simulink model "mdl"  (R2024a)
settings: Solver=ode1  StartTime=0.0  StopTime=inf  FixedStep=0.1  RelTol=1e-3  EnableMultiTasking=on
values from neighbouring files (symbols this model uses):
  A = 1    [init.m]
  Cw = 1.1    [init.m]
  fr = 0.02    [init.m]
  g = 9.81    [init.m]
  i1 = 74/9    (= 8.22222222222)    [init.m]
  i2 = 58/10    (= 5.8)    [init.m]
  Jachse_mitte = 0.003    [init.m]
  Jachse_unten = 0.052    [init.m]
  Jmotor = 0.001    [init.m]
  Jrad = 0.2    [init.m]
  Kp = 4000    [init.m]
  m = 455    [init.m]
  m_achse_mitte = Jachse_mitte * i2*i2 / (rR*rR)    (= 1.70347629346)    [init.m]
  m_achse_unten = Jachse_unten / (rR*rR)    (= 0.877732533291)    [init.m]
  m_motor = Jmotor * i1*i1*i2*i2 / (rR*rR)    (= 38.3878032221)    [init.m]
  m_raeder = 4 * Jrad / (rR*rR)    (= 13.5035774353)    [init.m]
  rho = 1.2    [init.m]
  rR = 0.2434    [init.m]
  stop_distance = 10.6182    [init.m]
  Tn = 200    [init.m]
undefined symbols (not defined in the file or in its folder): gradient_distance_lookup, gradient_lookup
settings Model: Creator=roustiam  LastModifiedBy=Nico Hörter
settings SolverCC: AlgebraicLoopSolver=TrustRegion
settings DataIOCC: LimitDataPoints=on  SaveFormat=Array  SignalLoggingSaveFormat=ModelDataLogs  ReturnWorkspaceOutputs=off  SignalLoggingName=sigsOut
settings OptimizationCC: BlockReduction=off  BooleanDataType=off  ExpressionDepthLimit=2147483647  InitFltsAndDblsToZero=on  LifeSpan=inf
settings DebuggingCC: SaveWithParameterizedLinksMsg=none  UnderspecifiedInitializationDetection=Classic  MergeDetectMultiDrivingBlocksExec=none  SignalResolutionControl=TryResolveAllWithWarning  MultiTaskDSMMsg=warning  MultiTaskCondExecSysMsg=none  FcnCallInpInsideContextMsg=warning  UnconnectedInputMsg=warning  UnconnectedOutputMsg=warning  UnconnectedLineMsg=warning  StateNameClashWarn=warning  SFUnexpectedBacktrackingDiag=warning  SFNoUnconditionalDefaultTransitionDiag=warning  ArithmeticOperatorsInVariantConditions=warning
settings HardwareCC: ProdBitPerPointer=32  ProdBitPerSizeT=32  ProdBitPerPtrDiffT=32  ProdLargestAtomicFloat=None  ProdIntDivRoundTo=Undefined  ProdEndianess=Unspecified  ProdWordSize=32  ProdHWDeviceType=32-bit Generic  TargetUnknown=on
settings ModelReferenceCC: EnableRefExpFcnMdlSchedulingChecks=on  PropagateSignalLabelsOutOfModel=off
settings SFSimCC: SimUseLocalCustomCode=off  CustomCodeUndefinedFunction=UseInterfaceOnly
settings RTWCC: RTWUseLocalCustomCode=off  GPUComputeCapability=3.5
settings CodeAppCC: StateflowObjectComments=on
settings GRTTargetCC: TargetFcnLib=ansi_tfl_tmw.mat  TargetLangStandard=C89/C90 (ANSI)  CombineOutputUpdateFcns=off  GRTInterface=on
settings ConfigComp: CovMetricSettings=dw  CovSaveCumulativeToWorkspaceVar=on  CovSaveSingleToWorkspaceVar=on  CovExternalEMLEnable=off

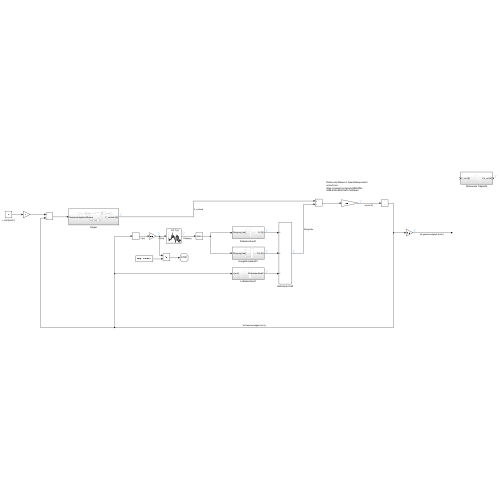
[thumbnail: Simulink's stored preview of the top-level diagram]
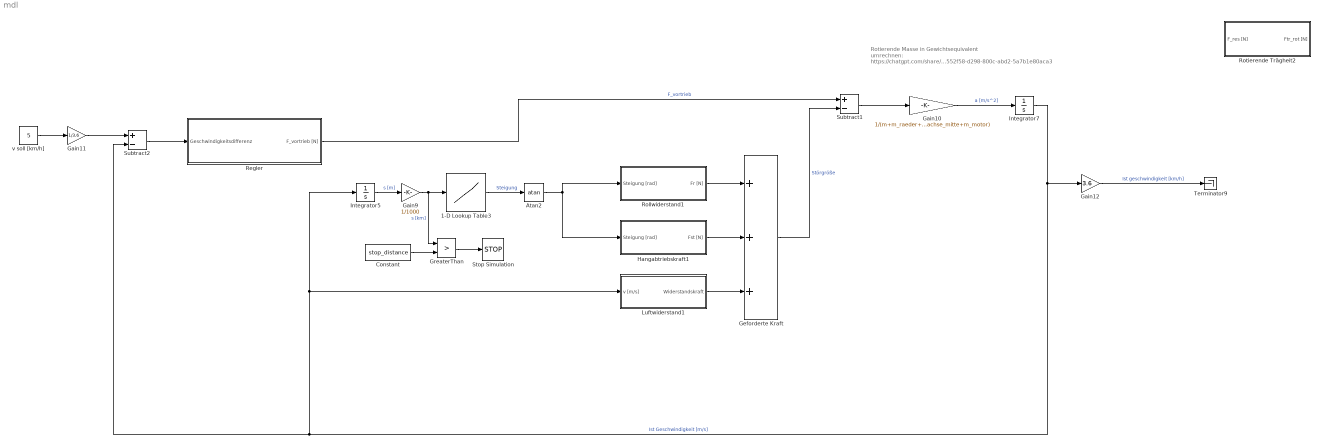
== system mdl ==
  note: Rotierende Masse in Gewichtsequivalent umrechnen:
      | https://chatgpt.com/share/68552f58-d298-800c-abd2-5a7b1e80aca3
  1-D Lookup Table3 : Lookup_n-D  NumberOfTableDimensions=1  BreakpointsForDimension1=gradient_distance_lookup  Table=gradient_lookup  ExtrapMethod=Clip  InternalRulePriority=Speed  RndMeth=Simplest
  Atan2 : Trigonometry  Operator=atan
  Constant : Constant  Value=stop_distance
  Gain10 : Gain  Gain=1/(m+m_raeder+m_achse_unten+m_achse_mitte+m_motor)
  Gain11 : Gain  Gain=1/3.6
  Gain12 : Gain  Gain=3.6
  Gain9 : Gain  Gain=1/1000
  Geforderte Kraft : Sum  Inputs=+++
  GreaterThan : RelationalOperator  Operator=>  OutDataTypeStr=boolean  RndMeth=Simplest  InputSameDT=off
  Hangabtriebskraft1 : Subsystem
  Integrator5 : Integrator
  Integrator7 : Integrator
  Luftwiderstand1 : Subsystem
  Regler : Subsystem
  Rollwiderstand1 : Subsystem
  Rotierende Trägheit2 : Subsystem
  Stop Simulation : Stop
  Subtract1 : Sum  Inputs=+-
  Subtract2 : Sum  Inputs=+-
  Terminator9 : Terminator
  v soll [km/h] : Constant  Value=5
  wires:
  Atan2/1 -> Rollwiderstand1/1(Steigung [rad]), Hangabtriebskraft1/1(Steigung [rad])
  1-D Lookup Table3/1 -> Atan2/1  "Steigung"
  Gain9/1 -> GreaterThan/1, 1-D Lookup Table3/1  "s [km]"
  Integrator5/1 -> Gain9/1  "s [m]"
  Rollwiderstand1/1(Fr [N]) -> Geforderte Kraft/1
  Hangabtriebskraft1/1(Fst [N]) -> Geforderte Kraft/2
  Luftwiderstand1/1(Widerstandskraft) -> Geforderte Kraft/3
  Gain10/1 -> Integrator7/1  "a [m/s^2]"
  Integrator7/1 -> Gain12/1, Integrator5/1, Luftwiderstand1/1(v [m/s]), Subtract2/2  "Ist Geschwindigkeit [m/s]"
  Geforderte Kraft/1 -> Subtract1/2  "Störgröße"
  Regler/1(F_vortrieb [N]) -> Subtract1/1  "F_vortrieb"
  Subtract1/1 -> Gain10/1
  v soll [km/h]/1 -> Gain11/1
  Gain11/1 -> Subtract2/1
  Subtract2/1 -> Regler/1(Geschwindigkeitsdifferenz)
  Gain12/1 -> Terminator9/1  "Ist geschwindigkeit [km/h]"
  GreaterThan/1 -> Stop Simulation/1
  Constant/1 -> GreaterThan/2

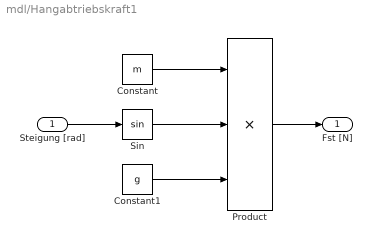
== system mdl/Hangabtriebskraft1 ==
  Steigung [rad] : Inport
  Constant : Constant  Value=m
  Constant1 : Constant  Value=g
  Product : Product  Inputs=3
  Sin : Trigonometry
  Fst [N] : Outport
  wires:
  Product/1 -> Fst [N]/1
  Constant/1 -> Product/1
  Sin/1 -> Product/2
  Steigung [rad]/1 -> Sin/1
  Constant1/1 -> Product/3

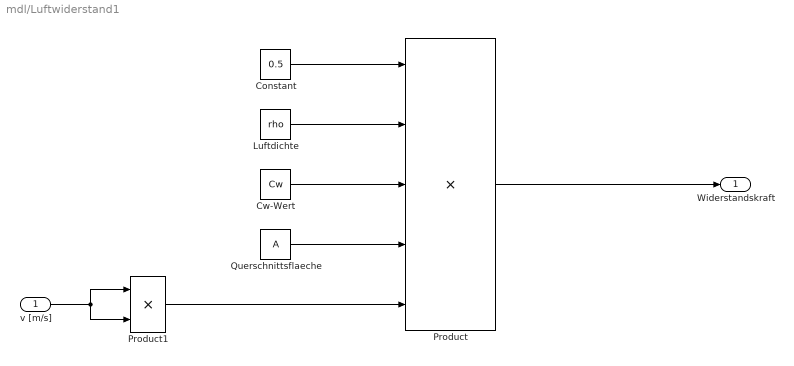
== system mdl/Luftwiderstand1 ==
  v [m/s] : Inport
  Constant : Constant  Value=0.5
  Cw-Wert : Constant  Value=Cw
  Luftdichte : Constant  Value=rho
  Product : Product  Inputs=5
  Product1 : Product
  Querschnittsflaeche : Constant  Value=A
  Widerstandskraft : Outport
  wires:
  Querschnittsflaeche/1 -> Product/4
  Cw-Wert/1 -> Product/3
  Luftdichte/1 -> Product/2
  Constant/1 -> Product/1
  Product1/1 -> Product/5
  v [m/s]/1 -> Product1/1, Product1/2
  Product/1 -> Widerstandskraft/1

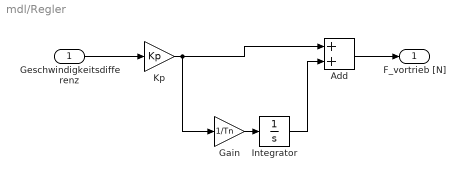
== system mdl/Regler ==
  Geschwindigkeitsdifferenz : Inport
  Add : Sum
  Gain : Gain  Gain=1/Tn
  Integrator : Integrator
  Kp : Gain  Gain=Kp
  F_vortrieb [N] : Outport
  wires:
  Geschwindigkeitsdifferenz/1 -> Kp/1
  Add/1 -> F_vortrieb [N]/1
  Kp/1 -> Gain/1, Add/1
  Gain/1 -> Integrator/1
  Integrator/1 -> Add/2

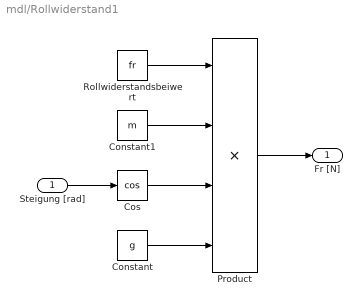
== system mdl/Rollwiderstand1 ==
  Steigung [rad] : Inport
  Constant : Constant  Value=g
  Constant1 : Constant  Value=m
  Cos : Trigonometry  Operator=cos
  Product : Product  Inputs=4
  Rollwiderstandsbeiwert : Constant  Value=fr
  Fr [N] : Outport
  wires:
  Steigung [rad]/1 -> Cos/1
  Product/1 -> Fr [N]/1
  Constant/1 -> Product/4
  Cos/1 -> Product/3
  Constant1/1 -> Product/2
  Rollwiderstandsbeiwert/1 -> Product/1

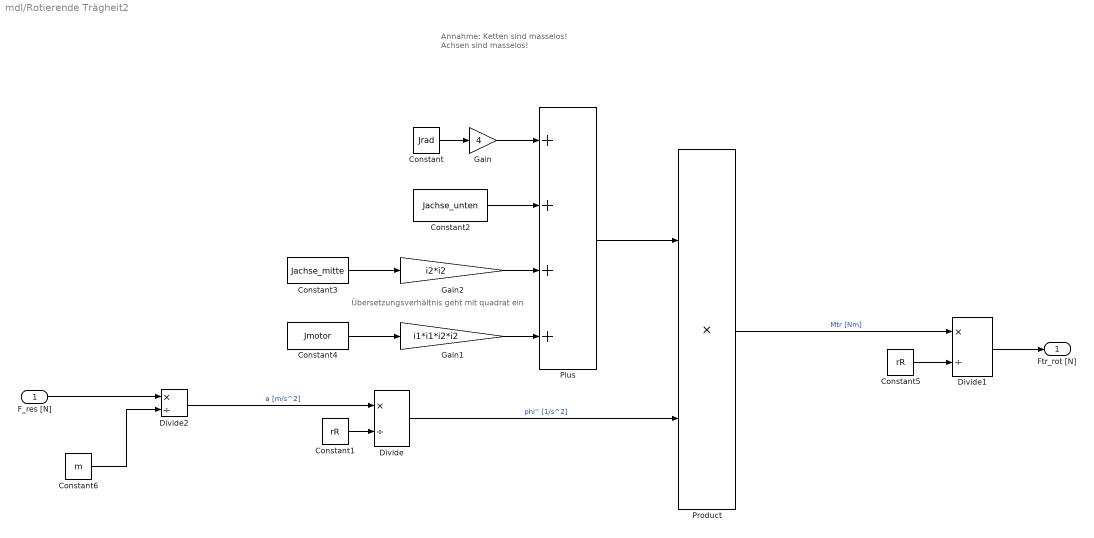
== system mdl/Rotierende Trägheit2 ==
  note: Übersetzungsverhältnis geht mit quadrat ein
  note: Annahme: Ketten sind masselos!
      | Achsen sind masselos!
  F_res [N] : Inport
  Constant : Constant  Value=Jrad
  Constant1 : Constant  Value=rR
  Constant2 : Constant  Value=Jachse_unten
  Constant3 : Constant  Value=Jachse_mitte
  Constant4 : Constant  Value=Jmotor
  Constant5 : Constant  Value=rR
  Constant6 : Constant  Value=m
  Divide : Product  Inputs=*/  RndMeth=Zero  SaturateOnIntegerOverflow=on
  Divide1 : Product  Inputs=*/
  Divide2 : Product  Inputs=*/
  Gain : Gain  Gain=4
  Gain1 : Gain  Gain=i1*i1*i2*i2
  Gain2 : Gain  Gain=i2*i2
  Plus : Sum  Inputs=++++
  Product : Product
  Ftr_rot [N] : Outport
  wires:
  Constant1/1 -> Divide/2
  Divide/1 -> Product/2  "phi'' [1/s^2]"
  Constant/1 -> Gain/1
  Gain/1 -> Plus/1
  Constant2/1 -> Plus/2
  Plus/1 -> Product/1
  Product/1 -> Divide1/1  "Mtr [Nm]"
  Constant4/1 -> Gain1/1
  Constant3/1 -> Gain2/1
  Gain2/1 -> Plus/3
  Gain1/1 -> Plus/4
  Constant5/1 -> Divide1/2
  Divide1/1 -> Ftr_rot [N]/1
  Divide2/1 -> Divide/1  "a [m/s^2]"
  F_res [N]/1 -> Divide2/1
  Constant6/1 -> Divide2/2
